simulink model "controlMCUSlugsMKII"  (Simulink 6.6)
settings: Solver=FixedStepDiscrete  StartTime=0.0  StopTime=10.0  FixedStep=0.01  RelTol=1e-3
InitFcn:
  | mcuInit
values from neighbouring files (symbols this model uses):
  apSampleTime = 0.01    [mcuInit.m]
  derivativesConstant = 5    [mcuInit.m]
  T = 0.01    [mcuInit.m]
undefined symbols (not defined in the file or in its folder): bankCommandLimit, baseHeight, bda, bde, bdr, bdt, bICda, bICde, bICdr, bICdt, controlMCUInit, daLimit, deLimit, drLimit, dtLimit, getAccBias, getAccels, getAttitude, getMidLevelCommands, getPassValues, getPidIdx, getVned, getWP, getXYZ, gsRead, ISA_g, lowRateTelemetryMavlink, mda, mde, mdr, mdt, mICda, mICde, mICdr, mICdt, pitchCommandLimit, protDecodeMavlink, readIpc, send2GS, setCurrentCommands, setDiagnosticFloat, setDiagnosticShort, setLogFloat1, setLogFloat2, setNavLat, setNavLong, setNavNav, u1, u2, updateEuler, updateLoad, updatePQR, updatePWM, updatePWM2, y1
libraries: dsPICdrivers x85, simulink x79, SLUGS_Library x23, aerolibconvert2 x5, aerolibutil x3
(part 2 of 5)

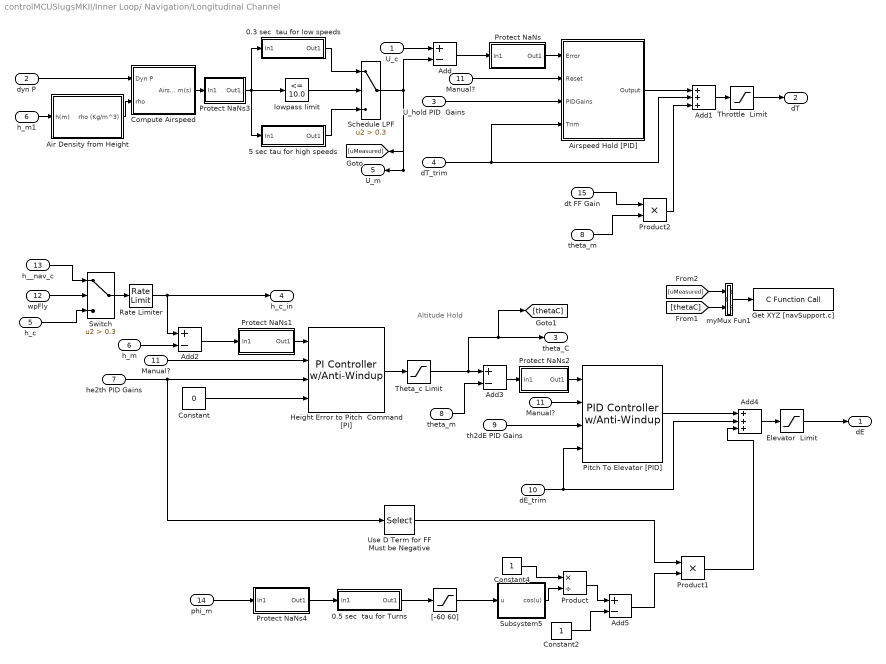
== system controlMCUSlugsMKII/Inner Loop/ Navigation/Longitudinal Channel ==
  note: Altitude Hold
  U_c : Inport
  dyn P : Inport  Port=2
  U_hold PID  Gains : Inport  Port=3
  dT_trim : Inport  Port=4
  h_c : Inport  Port=5
  h_m : Inport  Port=6
  he2th PID Gains : Inport  Port=7
  theta_m : Inport  Port=8
  th2dE PID Gains : Inport  Port=9
  dE_trim : Inport  Port=10
  Manual? : Inport  Port=11
  wpFly : Inport  Port=12  SampleTime=apSampleTime
  h__nav_c : Inport  Port=13
  phi_m : Inport  Port=14
  dt FF Gain : Inport  Port=15
  0.3 sec  tau for low speeds : Subsystem  mask(Tustin1stOrderLowpassAutoInitialCondition){f=0.5, T=T}
      mask prompts: f "Lowpass Frequency"; T "Sample Time"
      mask help: Takes a 3db rolloff frequency (in Hz, NOT radians/s) and a sample time. Performs a symbolic Tustin conversion and implements in a discrete filter. The initial output of the filter is set by the first sample.
      mask Help: Enter the desired 3db rolloff frequency in Hz and the sample time. Initial conditions are sampled automatically.
      mask Display: fprintf('%.2f Hz lowpass',f)
  0.5 sec  tau for Turns : Subsystem  mask(Tustin1stOrderLowpassAutoInitialCondition){f=0.32, T=T}
      mask prompts: f "Lowpass Frequency"; T "Sample Time"
      mask help: Takes a 3db rolloff frequency (in Hz, NOT radians/s) and a sample time. Performs a symbolic Tustin conversion and implements in a discrete filter. The initial output of the filter is set by the first sample.
      mask Help: Enter the desired 3db rolloff frequency in Hz and the sample time. Initial conditions are sampled automatically.
      mask Display: fprintf('%.2f Hz lowpass',f)
  5 sec tau for high speeds : Subsystem  mask(Tustin1stOrderLowpassAutoInitialCondition){f=.032, T=T}
      mask prompts: f "Lowpass Frequency"; T "Sample Time"
      mask help: Takes a 3db rolloff frequency (in Hz, NOT radians/s) and a sample time. Performs a symbolic Tustin conversion and implements in a discrete filter. The initial output of the filter is set by the first sample.
      mask Help: Enter the desired 3db rolloff frequency in Hz and the sample time. Initial conditions are sampled automatically.
      mask Display: fprintf('%.2f Hz lowpass',f)
  Add : Sum  Inputs=+-  OutScaling=2^-10
  Add1 : Sum  Inputs=3  OutDataTypeMode=single  OutScaling=2^-10
  Add2 : Sum  Inputs=+-  OutDataTypeMode=single  OutScaling=2^-10
  Add3 : Sum  Inputs=+-  OutDataTypeMode=single  OutScaling=2^-10
  Add4 : Sum  Inputs=3  OutDataTypeMode=single  OutScaling=2^-10
  Add5 : Sum  Inputs=+-  OutDataTypeMode=single  OutScaling=2^-10
  Air Density from Height : Subsystem  AncestorBlock=SLUGS_Library/Air Density from Height
  Airspeed Hold [PID] : Subsystem  AncestorBlock=SLUGS_Library/Control Blocks/PID Controller w//Anti-Windup  mask(PID){Tsample=apSampleTime, Ndelay=derivativesConstant, upperSaturationLimit=dtLimit, lowerSaturationLimit=0}
      mask prompts: Tsample "Sample Time"; Ndelay "Integer delays for de/dt"; upperSaturationLimit "Upper Saturation Limit"; lowerSaturationLimit "Lower Saturation Limit"
      mask help: PID controller block with anti-windup and saturation limits. Implemented as a discrete forwardl integration which stops integrating when the output is saturated. Derivative is implemented as a numerical derivative with N integer delays to smooth output.
      mask Display:
      | disp('PID')
      | port_label('input',1,'error')
      | port_label('input',3,'gains')
      | port_label('input',2,'reset')
      | port_label('input',4,'trim')
      | port_label('output',1,'output')
  Compute Airspeed : Subsystem  AncestorBlock=SLUGS_Library/Compute Airspeed
  Constant : Constant  Value=0
  Constant2 : Constant  OutDataTypeMode=single
  Constant4 : Constant  OutDataTypeMode=single
  Elevator  Limit : Saturate  UpperLimit=deLimit  LowerLimit=-deLimit  SampleTime=apSampleTime
  Get XYZ [navSupport.c] : dsPICdrivers/OTHERS/C Function Call  Tag=dsPIC_dsPIC_CFunctionCall  fctName='setNavLong'  INPUT_SIZE=2  INPUT1=real32  INPUT2=--  INPUT3=--  OUTPUT_SIZE=1  OUTPUT1=--  SampleTime=.01  InputType=[ 7 ]  OutputType=[ ]  FctDeclaration=extern void setNavLong(real32_T* u1);  FctCall=setNavLong(*%u1);  OrderingInOutPopup=None
  Height Error to Pitch  Command [PI] : SLUGS_Library/Control Blocks/PI Controller w//Anti-Windup  SystemSampleTime=-1  Tsample=apSampleTime  Ndelay=derivativesConstant  upperSaturationLimit=pitchCommandLimit  lowerSaturationLimit=-pitchCommandLimit
  "Manual? " : InportShadow  Port=11  LatchByCopyingInsideSignal=off
  "Manual?  " : InportShadow  Port=11  LatchByCopyingInsideSignal=off
  Pitch To Elevator [PID] : SLUGS_Library/Control Blocks/PID Controller w//Anti-Windup  SystemSampleTime=-1  Tsample=apSampleTime  Ndelay=derivativesConstant  upperSaturationLimit=deLimit  lowerSaturationLimit=-deLimit
  Product : Product  Inputs=*/  RndMeth=Zero
  Product1 : Product  RndMeth=Zero
  Product2 : Product  RndMeth=Zero
  Protect NaNs : Subsystem
  Protect NaNs1 : Subsystem
  Protect NaNs2 : Subsystem
  Protect NaNs3 : Subsystem
  Protect NaNs4 : Subsystem
  Rate Limiter : RateLimiter  RisingSlewLimit=7  FallingSlewLimit=-5  SampleTimeMode=inherited  InitialCondition=baseHeight
  Schedule LPF : Switch  Criteria=u2 > Threshold  Threshold=0.3
  Subsystem5 : Subsystem  AncestorBlock=SLUGS_Library/Subsystem5
  Switch : Switch  Criteria=u2 > Threshold  Threshold=0.3  InputSameDT=on
  Theta_c Limit : Saturate  UpperLimit=pitchCommandLimit  LowerLimit=-pitchCommandLimit  SampleTime=apSampleTime
  Throttle  Limit : Saturate  UpperLimit=dtLimit  LowerLimit=0  SampleTime=apSampleTime
  Use D Term for FF Must be Negative : Selector  IndexOptions=Index vector (dialog)  Indices=3  OutputSizes=1  InputPortWidth=3
  "[-60 60]" : Saturate  UpperLimit=60  LowerLimit=-60  SampleTime=apSampleTime
  h_m1 : InportShadow  Port=6  LatchByCopyingInsideSignal=off
  lowpass limit : simulink/Logic and Bit Operations/Compare To Constant  SystemSampleTime=-1  relop=<=  const=10.0  LogicOutDataTypeMode=uint8  ZeroCross=off
  myMux Fun1 : Stateflow chart
  "theta_m " : InportShadow  Port=8  LatchByCopyingInsideSignal=off
  dE : Outport
  dT : Outport  Port=2
  theta_C : Outport  Port=3
  h_c_in : Outport  Port=4
  U_m : Outport  Orientation=left  Port=5
  wires:
  Height Error to Pitch  Command [PI]/1 -> Theta_c Limit/1
  Rate Limiter/1 -> Add2/1, h_c_in/1
  h__nav_c/1 -> Switch/1
  h_c/1 -> Switch/3
  Switch/1 -> Rate Limiter/1
  wpFly/1 -> Switch/2
  Theta_c Limit/1 -> Add3/1, theta_C/1, [thetaC]
  Add3/1 -> Protect NaNs2/1(In1)
  th2dE PID Gains/1 -> Pitch To Elevator [PID]/3
  he2th PID Gains/1 -> Use D Term for FF Must be Negative/1, Height Error to Pitch  Command [PI]/3
  h_m1/1 -> Air Density from Height/1(h(m))
  dyn P/1 -> Compute Airspeed/1(Dyn P)
  Air Density from Height/1(rho (Kg/m^3)) -> Compute Airspeed/2(rho)
  Elevator  Limit/1 -> dE/1
  dE_trim/1 -> Add4/2, Pitch To Elevator [PID]/4
  Pitch To Elevator [PID]/1 -> Add4/1
  Add4/1 -> Elevator  Limit/1
  "Manual?  "/1 -> Pitch To Elevator [PID]/2
  "Manual? "/1 -> Height Error to Pitch  Command [PI]/2
  Manual?/1 -> Airspeed Hold [PID]/2(Reset)
  theta_m/1 -> Add3/2
  h_m/1 -> Add2/2
  Add2/1 -> Protect NaNs1/1(In1)
  Throttle  Limit/1 -> dT/1
  Add1/1 -> Throttle  Limit/1
  dT_trim/1 -> Add1/2, Airspeed Hold [PID]/4(Trim)
  Airspeed Hold [PID]/1(Output) -> Add1/1
  Add/1 -> Protect NaNs/1(In1)
  U_c/1 -> Add/1
  myMux Fun1/1(y) -> Get XYZ [navSupport.c]/1
  [uMeasured] -> myMux Fun1/1(u1)
  [thetaC] -> myMux Fun1/2(u2)
  Schedule LPF/1 -> Add/2, U_m/1, [uMeasured]
  Compute Airspeed/1(Airspeed m(s)) -> Protect NaNs3/1(In1)
  lowpass limit/1 -> Schedule LPF/2
  5 sec tau for high speeds/1(Out1) -> Schedule LPF/3
  0.3 sec  tau for low speeds/1(Out1) -> Schedule LPF/1
  phi_m/1 -> Protect NaNs4/1(In1)
  Constant2/1 -> Add5/2
  Subsystem5/1(cos(u)) -> Product/2
  Constant4/1 -> Product/1
  Product/1 -> Add5/1
  0.5 sec  tau for Turns/1(Out1) -> "[-60 60]"/1
  "[-60 60]"/1 -> Subsystem5/1(u)
  Add5/1 -> Product1/2
  Use D Term for FF Must be Negative/1 -> Product1/1
  Product1/1 -> Add4/3
  "theta_m "/1 -> Product2/2
  Product2/1 -> Add1/3
  dt FF Gain/1 -> Product2/1
  U_hold PID  Gains/1 -> Airspeed Hold [PID]/3(PIDGains)
  Constant/1 -> Height Error to Pitch  Command [PI]/4
  Protect NaNs/1(Out1) -> Airspeed Hold [PID]/1(Error)
  Protect NaNs1/1(Out1) -> Height Error to Pitch  Command [PI]/1
  Protect NaNs2/1(Out1) -> Pitch To Elevator [PID]/1
  Protect NaNs3/1(Out1) -> 0.3 sec  tau for low speeds/1(In1), 5 sec tau for high speeds/1(In1), lowpass limit/1
  Protect NaNs4/1(Out1) -> 0.5 sec  tau for Turns/1(In1)

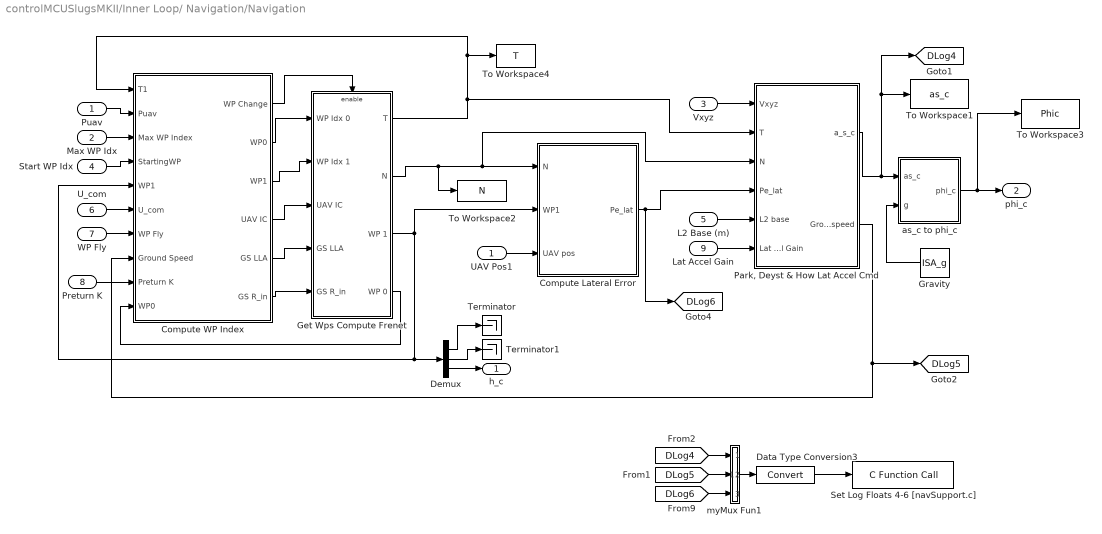
== system controlMCUSlugsMKII/Inner Loop/ Navigation/Navigation ==
  Puav : Inport  SampleTime=apSampleTime
  Max WP Idx : Inport  Port=2
  Vxyz : Inport  Port=3
  Start WP Idx : Inport  Port=4
  L2 Base (m) : Inport  Port=5
  U_com : Inport  Port=6
  WP Fly : Inport  Port=7
  Preturn K : Inport  Port=8
  Lat Accel Gain : Inport  Port=9
  Compute Lateral Error : Subsystem  AncestorBlock=SLUGS_Library/Navigation/Compute Lateral Error
  Compute WP Index : Subsystem
  Data Type Conversion3 : DataTypeConversion  OutDataTypeMode=single
  Demux : Demux  Outputs=3
  Get Wps Compute Frenet : Subsystem
  Gravity : Constant  Orientation=left  Value=ISA_g  OutDataTypeMode=single
  "Park, Deyst & How Lat Accel Cmd" : Subsystem  AncestorBlock=SLUGS_Library/Navigation/Park, Deyst & How Lat Accel Cmd
  Set Log Floats 4-6 [navSupport.c] : dsPICdrivers/OTHERS/C Function Call  Tag=dsPIC_dsPIC_CFunctionCall  fctName='setLogFloat2'  INPUT_SIZE=3  INPUT1=real32  INPUT2=--  INPUT3=--  OUTPUT_SIZE=1  OUTPUT1=--  SampleTime=.01  InputType=[ 7 ]  OutputType=[ ]  FctDeclaration=extern void setLogFloat2(real32_T* u1);  FctCall=setLogFloat2(*%u1);  OrderingInOutPopup=None
  Terminator : Terminator
  Terminator1 : Terminator
  To Workspace1 : ToWorkspace  VariableName=as_c  SampleTime=-1  SaveFormat=Array
  To Workspace2 : ToWorkspace  VariableName=N  SampleTime=-1  SaveFormat=Array
  To Workspace3 : ToWorkspace  VariableName=Phic  SampleTime=-1  SaveFormat=Array
  To Workspace4 : ToWorkspace  VariableName=T  SampleTime=-1  SaveFormat=Array
  UAV Pos1 : InportShadow  Port=1  SampleTime=apSampleTime  LatchByCopyingInsideSignal=off
  as_c to phi_c : Subsystem  AncestorBlock=SLUGS_Library/Navigation/as_c to phi_c
  myMux Fun1 : Stateflow chart
  h_c : Outport
  phi_c : Outport  Port=2
  tag scope: DLog4=global, DLog5=global, DLog6=global
  wires:
  Demux/2 -> Terminator1/1
  Demux/1 -> Terminator/1
  Demux/3 -> h_c/1
  Compute WP Index/6(GS R_in) -> Get Wps Compute Frenet/5(GS R_in)
  Compute WP Index/5(GS LLA) -> Get Wps Compute Frenet/4(GS LLA)
  Compute WP Index/2(WP0) -> Get Wps Compute Frenet/1(WP Idx 0)
  Compute WP Index/3(WP1) -> Get Wps Compute Frenet/2(WP Idx 1)
  Get Wps Compute Frenet/2(N) -> Compute Lateral Error/1(N), "Park, Deyst & How Lat Accel Cmd"/3(N), To Workspace2/1
  Get Wps Compute Frenet/1(T) -> To Workspace4/1, Compute WP Index/1(T1), "Park, Deyst & How Lat Accel Cmd"/2(T)
  Puav/1 -> Compute WP Index/2(Puav)
  Max WP Idx/1 -> Compute WP Index/3(Max WP Index)
  Start WP Idx/1 -> Compute WP Index/4(StartingWP)
  "Park, Deyst & How Lat Accel Cmd"/1(a_s_c) -> as_c to phi_c/1(as_c), To Workspace1/1, [DLog4]
  UAV Pos1/1 -> Compute Lateral Error/3(UAV pos)
  as_c to phi_c/1(phi_c) -> phi_c/1, To Workspace3/1
  Gravity/1 -> as_c to phi_c/2(g)
  Compute Lateral Error/1(Pe_lat) -> "Park, Deyst & How Lat Accel Cmd"/4(Pe_lat), [DLog6]
  Get Wps Compute Frenet/3(WP 1) -> Compute Lateral Error/2(WP1), Demux/1, Compute WP Index/5("WP1 ")
  L2 Base (m)/1 -> "Park, Deyst & How Lat Accel Cmd"/5(L2 base)
  Compute WP Index/1(WP Change) -> Get Wps Compute Frenet/Enable
  U_com/1 -> Compute WP Index/6(U_com)
  Vxyz/1 -> "Park, Deyst & How Lat Accel Cmd"/1(Vxyz)
  WP Fly/1 -> Compute WP Index/7(WP Fly)
  Compute WP Index/4(UAV IC) -> Get Wps Compute Frenet/3(UAV IC)
  "Park, Deyst & How Lat Accel Cmd"/2(Groundspeed) -> Compute WP Index/8(Ground Speed), [DLog5]
  Preturn K/1 -> Compute WP Index/9(Preturn K)
  Get Wps Compute Frenet/4(WP 0) -> Compute WP Index/10("WP0 ")
  Lat Accel Gain/1 -> "Park, Deyst & How Lat Accel Cmd"/6(Lat Accel Gain)
  [DLog4] -> myMux Fun1/1(u1)
  [DLog5] -> myMux Fun1/2(u2)
  [DLog6] -> myMux Fun1/3(u3)
  myMux Fun1/1(y) -> Data Type Conversion3/1
  Data Type Conversion3/1 -> Set Log Floats 4-6 [navSupport.c]/1

== system controlMCUSlugsMKII/Inner Loop/ Navigation/Protect NaNs ==
  In1 : Inport
  Integer Delay3 : simulink/Discrete/Integer Delay  Orientation=left  vinit=0.0  samptime=T  NumDelays=1
  Relational Operator2 : RelationalOperator  Operator===  LogicOutDataTypeMode=Specify via dialog
  Switch3 : Switch  Criteria=u2 > Threshold  Threshold=0.3  SampleTime=.01
  Out1 : Outport  Orientation=down
  wires:
  Integer Delay3/1 -> Switch3/3
  Switch3/1 -> Out1/1, Integer Delay3/1
  In1/1 -> Relational Operator2/2, Relational Operator2/1, Switch3/1
  Relational Operator2/1 -> Switch3/2

== system controlMCUSlugsMKII/Trim Vals/Bufffer IC ==
  Pilot Console : Inport
  Buffer IC Channel : Stateflow chart
  Buffer IC Channel1 : Stateflow chart
  Buffer IC Channel2 : Stateflow chart
  Buffer IC Channel3 : Stateflow chart
  Demux : Demux
  dT_buf : Outport
  dA_buf : Outport  Port=2
  dR_buf : Outport  Port=3
  dE_buf : Outport  Port=4
  wires:
  Demux/1 -> Buffer IC Channel/1(latest)
  Demux/2 -> Buffer IC Channel1/1(latest)
  Demux/3 -> Buffer IC Channel2/1(latest)
  Demux/4 -> Buffer IC Channel3/1(latest)
  Pilot Console/1 -> Demux/1
  Buffer IC Channel/1(history) -> dT_buf/1
  Buffer IC Channel1/1(history) -> dA_buf/1
  Buffer IC Channel2/1(history) -> dR_buf/1
  Buffer IC Channel3/1(history) -> dE_buf/1

== system controlMCUSlugsMKII/Trim Vals/Control Surface Input ==
  Input Capture : dsPICdrivers/Peripheral I//O/Input Capture  Tag=dsPIC_PWM_IC  Priority=5  IntPriority=6  Channel=[ 2 3 4 5 8]  Channel_UP_Down_Periode="[1  1  1  1  1]"  MaxChannel="[0.0025      0.0025      0.0025      0.0025      0.0025]"  SafeMarge="[10  10  10  10  10]"  MaxName=' IC2max , IC3max , IC4max , IC5max , IC8max '  Precision="[13.7469      13.7469      13.7469      13.7469      13.7469]"  Timer="[2  2  2  2  2]"  ChangeDetected="[0  0  0  0  0]"  ChangeDetectedPortRef=3  SampleTime=.01  Status=OK
  myMux Fun5 : Stateflow chart
  Pilot Console : Outport
  wires:
  myMux Fun5/1(y) -> Pilot Console/1
  Input Capture/1 -> myMux Fun5/1(u1)
  Input Capture/2 -> myMux Fun5/2(u2)
  Input Capture/3 -> myMux Fun5/3(u3)
  Input Capture/4 -> myMux Fun5/4(u4)
  Input Capture/5 -> myMux Fun5/5(u5)

== system controlMCUSlugsMKII/Trim Vals/Detect Transition High to Low ==
  Switch : Inport
  Add : Sum  Orientation=left  Inputs=2  OutDataTypeMode=uint8  OutScaling=2^-10
  Data Type Conversion : DataTypeConversion  OutDataTypeMode=double  SampleTime=apSampleTime
  Hit  Crossing : HitCross  HitCrossingOffset=0.5  HitCrossingDirection=falling  SampleTime=apSampleTime
  IC : InitialCondition  Orientation=down
  Integer Delay2 : simulink/Discrete/Integer Delay  Orientation=left  vinit=0  samptime=-1  NumDelays=1
  Transition : Outport  Orientation=left
  wires:
  Hit  Crossing/1 -> IC/1
  Data Type Conversion/1 -> Hit  Crossing/1
  Integer Delay2/1 -> Add/1
  IC/1 -> Add/2, Integer Delay2/1
  Switch/1 -> Data Type Conversion/1
  Add/1 -> Transition/1

== system controlMCUSlugsMKII/Trim Vals/Grab I.C. ==
  dT_buf : Inport
  dA_buf : Inport  Port=2
  dR_buf : Inport  Port=3
  dE_buf : Inport  Port=4
  U_m : Inport  Port=5
  Enable : EnablePort
  Choose the Median [navSupport.c]{,1..3} (4 alike) : dsPICdrivers/OTHERS/C Function Call  Tag=dsPIC_dsPIC_CFunctionCall  fctName='meanFilter5'  INPUT_SIZE=7  INPUT1=uint16  INPUT2=--  INPUT3=--  OUTPUT_SIZE=1  OUTPUT1=uint16  SampleTime=.01  InputType=[ 4 ]  OutputType=[ 4 ]  FctDeclaration=extern uint16_T meanFilter5(uint16_T* u1);  FctCall=%y1 = meanFilter5(*%u1);  OrderingInOutPopup=None
  Convert to Rad : Subsystem  mask{slopem=mICdt, interceptb=bICdt}
      mask prompts: slopem "Slope"; interceptb "Intercept"
  Convert to Rad1 : Subsystem  mask{slopem=mICda, interceptb=bICda}
      mask prompts: slopem "Slope"; interceptb "Intercept"
  Convert to Rad2 : Subsystem  mask{slopem=mICdr, interceptb=bICdr}
      mask prompts: slopem "Slope"; interceptb "Intercept"
  Convert to Rad3 : Subsystem  mask{slopem=mICde, interceptb=bICde}
      mask prompts: slopem "Slope"; interceptb "Intercept"
  Set Current Height and Airspeed as Commands [navSupport.c] : dsPICdrivers/OTHERS/C Function Call  Tag=dsPIC_dsPIC_CFunctionCall  fctName='setCurrentCommands'  INPUT_SIZE=1  INPUT1=real32  INPUT2=--  INPUT3=--  OUTPUT_SIZE=1  OUTPUT1=--  SampleTime=.01  InputType=[ 7 ]  OutputType=[ ]  FctDeclaration=extern void setCurrentCommands(real32_T u1);  FctCall=setCurrentCommands(%u1);  OrderingInOutPopup=None
  dT_trim : Outport
  dA_trim : Outport  Port=2
  dR_trim : Outport  Port=3
  dE_trim : Outport  Port=4
  wires:
  U_m/1 -> Set Current Height and Airspeed as Commands [navSupport.c]/1
  Convert to Rad/1(Angle (rad)) -> dT_trim/1
  Convert to Rad1/1(Angle (rad)) -> dA_trim/1
  Convert to Rad2/1(Angle (rad)) -> dR_trim/1
  Convert to Rad3/1(Angle (rad)) -> dE_trim/1
  Choose the Median [navSupport.c]/1 -> Convert to Rad/1(IC)
  Choose the Median [navSupport.c]1/1 -> Convert to Rad1/1(IC)
  Choose the Median [navSupport.c]2/1 -> Convert to Rad2/1(IC)
  Choose the Median [navSupport.c]3/1 -> Convert to Rad3/1(IC)
  dT_buf/1 -> Choose the Median [navSupport.c]/1
  dA_buf/1 -> Choose the Median [navSupport.c]1/1
  dR_buf/1 -> Choose the Median [navSupport.c]2/1
  dE_buf/1 -> Choose the Median [navSupport.c]3/1

== system controlMCUSlugsMKII/Trim Vals/Log  Trims Using PWM High [groundStationDriver.c] ==
  In1 : Inport
  In2 : Inport  Port=2
  In3 : Inport  Port=3
  In4 : Inport  Port=4
  Data Type Conversion{1..4} (4 alike) : DataTypeConversion  OutDataTypeMode=uint16  SampleTime=apSampleTime
  Report Airspeed : Subsystem
  Update PWM  Commands1 [updateControlMcu.c] : dsPICdrivers/OTHERS/C Function Call  Tag=dsPIC_dsPIC_CFunctionCall  fctName='updatePWM2'  INPUT_SIZE=1  INPUT1=uint16  INPUT2=uint8  INPUT3=--  OUTPUT_SIZE=1  OUTPUT1=--  SampleTime=-1  InputType=[ 4 2 ]  OutputType=[ ]  FctDeclaration=extern void updatePWM2(uint16_T u1, uint8_T u2);  FctCall=updatePWM2(%u1, %u2);  OrderingInOutPopup=None
  Update PWM  Commands2 [updateControlMcu.c] : dsPICdrivers/OTHERS/C Function Call  Tag=dsPIC_dsPIC_CFunctionCall  fctName='updatePWM2'  INPUT_SIZE=1  INPUT1=uint16  INPUT2=uint8  INPUT3=--  OUTPUT_SIZE=1  OUTPUT1=--  SampleTime=-1  InputType=[ 4 2 ]  OutputType=[ ]  FctDeclaration=extern void updatePWM2(uint16_T u1, uint8_T u2);  FctCall=updatePWM2(%u1, %u2);  OrderingInOutPopup=None
  Update PWM  Commands3 [updateControlMcu.c] : dsPICdrivers/OTHERS/C Function Call  Tag=dsPIC_dsPIC_CFunctionCall  fctName='updatePWM2'  INPUT_SIZE=1  INPUT1=uint16  INPUT2=uint8  INPUT3=--  OUTPUT_SIZE=1  OUTPUT1=--  SampleTime=-1  InputType=[ 4 2 ]  OutputType=[ ]  FctDeclaration=extern void updatePWM2(uint16_T u1, uint8_T u2);  FctCall=updatePWM2(%u1, %u2);  OrderingInOutPopup=None
  Update PWM  Commands4 [updateControlMcu.c] : dsPICdrivers/OTHERS/C Function Call  Tag=dsPIC_dsPIC_CFunctionCall  fctName='updatePWM2'  INPUT_SIZE=1  INPUT1=uint16  INPUT2=uint8  INPUT3=--  OUTPUT_SIZE=1  OUTPUT1=--  SampleTime=-1  InputType=[ 4 2 ]  OutputType=[ ]  FctDeclaration=extern void updatePWM2(uint16_T u1, uint8_T u2);  FctCall=updatePWM2(%u1, %u2);  OrderingInOutPopup=None
  dlf : Constant  OutDataTypeMode=uint8
  dlf1 : Constant  Value=3  OutDataTypeMode=uint8
  dre : Constant  Value=0  OutDataTypeMode=uint8
  dre1 : Constant  Value=2  OutDataTypeMode=uint8
  wires:
  Data Type Conversion3/1 -> Update PWM  Commands2 [updateControlMcu.c]/1
  In2/1 -> Data Type Conversion3/1
  dlf/1 -> Update PWM  Commands2 [updateControlMcu.c]/2
  Data Type Conversion1/1 -> Update PWM  Commands3 [updateControlMcu.c]/1
  Data Type Conversion4/1 -> Update PWM  Commands4 [updateControlMcu.c]/1
  In3/1 -> Data Type Conversion1/1
  In4/1 -> Data Type Conversion4/1
  dre1/1 -> Update PWM  Commands3 [updateControlMcu.c]/2
  dlf1/1 -> Update PWM  Commands4 [updateControlMcu.c]/2
  Data Type Conversion2/1 -> Update PWM  Commands1 [updateControlMcu.c]/1
  dre/1 -> Update PWM  Commands1 [updateControlMcu.c]/2
  In1/1 -> Data Type Conversion2/1

== system controlMCUSlugsMKII/Update PWM Commands and Send Telemetry/Generate PWM Signals Based on the Control Type ==
  Ctrl Type : Inport
  PWM(rad) : Inport  Port=2
  Pilot Console (IC) : Inport  Port=3
  Data Type Conversion : DataTypeConversion  OutDataTypeMode=uint16
  If : If  IfExpression=u1 == 1  ElseIfExpressions=((u1 == 2 ) | (u1 == 3)), u1 == 4, u1 == 5  ShowElse=off  SampleTime=.01
  If  Control Type Is Manual : Subsystem  TreatAsAtomicUnit=on
  If  Control Type Is Passthrough : Subsystem  TreatAsAtomicUnit=on
  If  Control Type Is Selective Passthrough : Subsystem  TreatAsAtomicUnit=on
  If  Control Type Is Wp Follow  or Inner Cmds : Subsystem  TreatAsAtomicUnit=on
  Merge : Merge  Inputs=4
  PWM : Outport
  wires:
  If/1 -> If  Control Type Is Manual/Action
  If/2 -> If  Control Type Is Wp Follow  or Inner Cmds/Action
  If/3 -> If  Control Type Is Passthrough/Action
  If/4 -> If  Control Type Is Selective Passthrough/Action
  If  Control Type Is Manual/1(PWM) -> Merge/1
  If  Control Type Is Wp Follow  or Inner Cmds/1(PWM (abs)) -> Merge/2
  If  Control Type Is Passthrough/1(PWM (abs)) -> Merge/3
  If  Control Type Is Selective Passthrough/1(PWM) -> Merge/4
  PWM(rad)/1 -> If  Control Type Is Selective Passthrough/1(PWM(rad)), If  Control Type Is Wp Follow  or Inner Cmds/1(PWM(rad))
  Pilot Console (IC)/1 -> If  Control Type Is Passthrough/1(Pilot (IC)), If  Control Type Is Selective Passthrough/2(Pilot (IC)), If  Control Type Is Manual/1(Pilot (IC))
  Ctrl Type/1 -> If/1
  Merge/1 -> Data Type Conversion/1
  Data Type Conversion/1 -> PWM/1

== system controlMCUSlugsMKII/get Nav Vars/Direction Cosine Matrix to Euler Angles ==
  DCM : Inport  PortDimensions=[3,3]
  "Reshape 3x3 -> 9" : Reshape  OutputDimensions=[9, 1]
  Subsystem1 : Subsystem  AncestorBlock=SLUGS_Library/Subsystem4
  Subsystem2 : Subsystem  AncestorBlock=SLUGS_Library/Subsystem4
  Subsystem3 : Subsystem  AncestorBlock=SLUGS_Library/Subsystem6
  cos(phi)cos(theta) : Subsystem
  cos(psi)cos(theta) : Subsystem
  sin(phi)cos(theta) : Subsystem
  sin(psi)cos(theta) : Subsystem
  sin(theta) : Subsystem
  phi : Outport  PortDimensions=1  InitialOutput=0
  theta : Outport  Port=2  PortDimensions=1  InitialOutput=0
  psi : Outport  Port=3  PortDimensions=1  InitialOutput=0
  wires:
  DCM/1 -> "Reshape 3x3 -> 9"/1
  "Reshape 3x3 -> 9"/1 -> sin(theta)/1(DCM), cos(phi)cos(theta)/1(DCM), sin(phi)cos(theta)/1(DCM), cos(psi)cos(theta)/1(DCM), sin(psi)cos(theta)/1(DCM)
  sin(theta)/1(sin(theta)) -> Subsystem3/1(x)
  sin(phi)cos(theta)/1(sin(phi)cos(theta)) -> Subsystem2/1(u)
  cos(phi)cos(theta)/1(cos(phi)cos(theta)) -> Subsystem2/2(v)
  sin(psi)cos(theta)/1(sin(psi)cos(theta)) -> Subsystem1/1(u)
  cos(psi)cos(theta)/1(cos(psi)cos(theta)) -> Subsystem1/2(v)
  Subsystem2/1(atan2(x,y)) -> phi/1  "phi"
  Subsystem3/1(asin(x)) -> theta/1  "theta"
  Subsystem1/1(atan2(x,y)) -> psi/1  "psi"

== system controlMCUSlugsMKII/get Nav Vars/Euler Angles to  Direction Cosine Matrix1 ==
  Euler Roll Pitch Yaw : Inport  PortDimensions=3
  A11 : Subsystem
  A12 : Subsystem
  A13 : Subsystem
  A21 : Subsystem
  A22 : Subsystem
  A23 : Subsystem
  A31 : Subsystem
  A32 : Subsystem
  A33 : Subsystem
  Create Transformation Matrix : Subsystem  AncestorBlock=aerolibutil/Create 3x3 Matrix  mask(Create 3x3 Matrix){}
      mask help:
      | Create a 3-by-3 matrix from nine input values. Each input corresponds to an element of the matrix.
      |
      | For example, the input labeled A21 is the entry in the second row and first column of the matrix.
      mask init:
      | aeroicon('aeroblk');
      mask Help: web(asbhelp);
      mask Display:
      | port_label('input',1,'A_{11}','texmode','on');
      | port_label('input',2,'A_{12}','texmode','on');
      | port_label('input',3,'A_{13}','texmode','on');
      | port_label('input',4,'A_{21}','texmode','on');
      | port_label('input',5,'A_{22}','texmode','on');
      | port_label('input',6,'A_{23}','texmode','on');
      | port_label('input',7,'A_{31}','texmode','on');
      | port_label('input',8,'A_{32}','texmode','on');
      | port_label('input',9,'A_{33}','texmode','on');
      | port_label('output',1,'A','texmode','on');
  Mux : Mux  Inputs=2
  Subsystem5 : Subsystem  AncestorBlock=SLUGS_Library/Subsystem5
  DCM : Outport  PortDimensions=[3,3]  InitialOutput=0
  wires:
  Mux/1 -> A33/1(sin_cos), A32/1(sin_cos), A31/1(sin_cos), A23/1(sin_cos), A13/1(sin_cos), A11/1(sin_cos), A12/1(sin_cos), A21/1(sin_cos), A22/1(sin_cos)
  Euler Roll Pitch Yaw/1 -> Subsystem5/1(u)
  Subsystem5/2(cos(u)) -> Mux/2
  Subsystem5/1(sin(u)) -> Mux/1
  Create Transformation Matrix/1(Matrix) -> DCM/1
  A21/1(A21) -> Create Transformation Matrix/4(M21)
  A31/1(A31) -> Create Transformation Matrix/7(M31)
  A32/1(A32) -> Create Transformation Matrix/8(M32)
  A33/1(A33) -> Create Transformation Matrix/9(M33)
  A23/1(A23) -> Create Transformation Matrix/6(M23)
  A12/1(A12) -> Create Transformation Matrix/2(M12)
  A11/1(A11) -> Create Transformation Matrix/1(M11)
  A22/1(A22) -> Create Transformation Matrix/5(M22)
  A13/1(A13) -> Create Transformation Matrix/3(M13)

== system controlMCUSlugsMKII/get Nav Vars/Euler Angles to  Direction Cosine Matrix2 ==
  Euler Roll Pitch Yaw : Inport  PortDimensions=3
  A11 : Subsystem
  A12 : Subsystem
  A13 : Subsystem
  A21 : Subsystem
  A22 : Subsystem
  A23 : Subsystem
  A31 : Subsystem
  A32 : Subsystem
  A33 : Subsystem
  Create Transformation Matrix : Subsystem  AncestorBlock=aerolibutil/Create 3x3 Matrix  mask(Create 3x3 Matrix){}
      mask help:
      | Create a 3-by-3 matrix from nine input values. Each input corresponds to an element of the matrix.
      |
      | For example, the input labeled A21 is the entry in the second row and first column of the matrix.
      mask init:
      | aeroicon('aeroblk');
      mask Help: web(asbhelp);
      mask Display:
      | port_label('input',1,'A_{11}','texmode','on');
      | port_label('input',2,'A_{12}','texmode','on');
      | port_label('input',3,'A_{13}','texmode','on');
      | port_label('input',4,'A_{21}','texmode','on');
      | port_label('input',5,'A_{22}','texmode','on');
      | port_label('input',6,'A_{23}','texmode','on');
      | port_label('input',7,'A_{31}','texmode','on');
      | port_label('input',8,'A_{32}','texmode','on');
      | port_label('input',9,'A_{33}','texmode','on');
      | port_label('output',1,'A','texmode','on');
  Mux : Mux  Inputs=2
  Subsystem5 : Subsystem  AncestorBlock=SLUGS_Library/Subsystem5
  DCM : Outport  PortDimensions=[3,3]  InitialOutput=0
  wires:
  A13/1(A13) -> Create Transformation Matrix/3(M13)
  A22/1(A22) -> Create Transformation Matrix/5(M22)
  A11/1(A11) -> Create Transformation Matrix/1(M11)
  A12/1(A12) -> Create Transformation Matrix/2(M12)
  A23/1(A23) -> Create Transformation Matrix/6(M23)
  A33/1(A33) -> Create Transformation Matrix/9(M33)
  A32/1(A32) -> Create Transformation Matrix/8(M32)
  A31/1(A31) -> Create Transformation Matrix/7(M31)
  A21/1(A21) -> Create Transformation Matrix/4(M21)
  Create Transformation Matrix/1(Matrix) -> DCM/1
  Subsystem5/1(sin(u)) -> Mux/1
  Subsystem5/2(cos(u)) -> Mux/2
  Euler Roll Pitch Yaw/1 -> Subsystem5/1(u)
  Mux/1 -> A22/1(sin_cos), A21/1(sin_cos), A12/1(sin_cos), A11/1(sin_cos), A13/1(sin_cos), A23/1(sin_cos), A31/1(sin_cos), A32/1(sin_cos), A33/1(sin_cos)

== system controlMCUSlugsMKII/Inner Loop/ Navigation/Compute psi_dot_m/Protect NaNs ==
  In1 : Inport
  Integer Delay3 : simulink/Discrete/Integer Delay  Orientation=left  vinit=0.0  samptime=T  NumDelays=1
  Relational Operator2 : RelationalOperator  Operator===  LogicOutDataTypeMode=Specify via dialog
  Switch3 : Switch  Criteria=u2 > Threshold  Threshold=0.3  SampleTime=.01
  Out1 : Outport  Orientation=down
  wires:
  Integer Delay3/1 -> Switch3/3
  Switch3/1 -> Out1/1, Integer Delay3/1
  In1/1 -> Relational Operator2/2, Relational Operator2/1, Switch3/1
  Relational Operator2/1 -> Switch3/2

== system controlMCUSlugsMKII/Inner Loop/ Navigation/Compute psi_dot_m/Subsystem5 ==
  u : Inport
  Environment Controller1 : simulink/Signal Routing/Environment Controller  SystemSampleTime=-1
  Trigonometric Function : Trigonometry  Operator=cos
  "[apUtils.c]" : dsPICdrivers/OTHERS/C Function Call  Tag=dsPIC_dsPIC_CFunctionCall  fctName='myCos'  INPUT_SIZE=1  INPUT1=real32  INPUT2=--  INPUT3=--  OUTPUT_SIZE=1  OUTPUT1=real32  SampleTime=-1  InputType=[ 7 ]  OutputType=[ 7 ]  FctDeclaration=extern real32_T myCos(real32_T u1);  FctCall=%y1 = myCos(%u1);  OrderingInOutPopup=None
  cos(u) : Outport
  wires:
  Trigonometric Function/1 -> Environment Controller1/1
  "[apUtils.c]"/1 -> Environment Controller1/2
  Environment Controller1/1 -> cos(u)/1
  u/1 -> Trigonometric Function/1, "[apUtils.c]"/1

== system controlMCUSlugsMKII/Inner Loop/ Navigation/Compute psi_dot_m/Subsystem7 ==
  x : Inport
  Environment Controller : simulink/Signal Routing/Environment Controller  SystemSampleTime=-1
  Trigonometric Function : Trigonometry
  "[apUtils.c]" : dsPICdrivers/OTHERS/C Function Call  Tag=dsPIC_dsPIC_CFunctionCall  fctName='mySin'  INPUT_SIZE=1  INPUT1=real32  INPUT2=--  INPUT3=--  OUTPUT_SIZE=1  OUTPUT1=real32  SampleTime=-1  InputType=[ 7 ]  OutputType=[ 7 ]  FctDeclaration=extern real32_T mySin(real32_T u1);  FctCall=%y1 = mySin(%u1);  OrderingInOutPopup=None
  sin(x) : Outport
  wires:
  x/1 -> "[apUtils.c]"/1, Trigonometric Function/1
  Trigonometric Function/1 -> Environment Controller/1
  "[apUtils.c]"/1 -> Environment Controller/2
  Environment Controller/1 -> sin(x)/1

== system controlMCUSlugsMKII/Inner Loop/ Navigation/L1 Output Feedback Controller With  Projection Operator/Control  Law ==
  a : Inport
  u : Inport  Port=2
  Compute Coef : Subsystem
  Detect Change : Subsystem
  Divide : Product  OutScaling=2^-10  SampleTime=apSampleTime
  Divide1 : Product  OutScaling=2^-10  SampleTime=apSampleTime
  IC : InitialCondition
  Integer Delay : simulink/Discrete/Integer Delay  vinit=0.0  samptime=apSampleTime  NumDelays=1
  Integer Delay1 : simulink/Discrete/Integer Delay  Orientation=left  vinit=0.0  samptime=apSampleTime  NumDelays=1
  Subtract : Sum  OutScaling=2^-10  SampleTime=apSampleTime
  y : Outport
  wires:
  a/1 -> Compute Coef/1(a), Detect Change/1(Data)
  Compute Coef/1(b) -> Divide/1
  Compute Coef/2(c) -> Divide1/1
  Detect Change/1(change?) -> IC/1
  Integer Delay/1 -> Divide/2
  Divide/1 -> Subtract/1
  Divide1/1 -> Subtract/2
  Subtract/1 -> y/1, Integer Delay1/1
  IC/1 -> Compute Coef/Enable
  u/1 -> Integer Delay/1
  Integer Delay1/1 -> Divide1/2

== system controlMCUSlugsMKII/Inner Loop/ Navigation/L1 Output Feedback Controller With  Projection Operator/Projection Operator ==
  Theta Max : Inport
  Eps 0 : Inport  Port=2
  Theta : Inport  Port=3
  y : Inport  Port=4
  Compare To Zero : simulink/Logic and Bit Operations/Compare To Zero  SystemSampleTime=-1  relop=>=  LogicOutDataTypeMode=boolean  ZeroCross=off
  Compare To Zero1 : simulink/Logic and Bit Operations/Compare To Zero  SystemSampleTime=-1  relop=>  LogicOutDataTypeMode=boolean  ZeroCross=off
  Divide2 : Product  OutDataTypeMode=single  OutScaling=2^-10
  Enabled Subsystem : Subsystem  TreatAsAtomicUnit=on
  Enabled Subsystem1 : Subsystem  TreatAsAtomicUnit=on
  F(theta) : Subsystem
  Logical Operator : Logic  Operator=NOT  AllPortsSameDT=off  OutDataTypeMode=Specify via dialog
  Logical Operator2 : Logic  Orientation=down  AllPortsSameDT=off  OutDataTypeMode=Specify via dialog
  Merge : Merge  InitialOutput=0
  "y " : InportShadow  Port=4  LatchByCopyingInsideSignal=off
  "y    " : InportShadow  Port=4  LatchByCopyingInsideSignal=off
  "Proj(the, y)" : Outport
  wires:
  Theta Max/1 -> F(theta)/1(Theta Max)
  Eps 0/1 -> F(theta)/2(Eps 0)
  Theta/1 -> F(theta)/3(Theta)
  F(theta)/1(f_theta) -> Compare To Zero/1, Enabled Subsystem1/2(f_the)
  y/1 -> Divide2/2
  Divide2/1 -> Compare To Zero1/1
  Merge/1 -> "Proj(the, y)"/1
  "y "/1 -> Enabled Subsystem/1(In1)
  Enabled Subsystem/1(Out1) -> Merge/1
  Compare To Zero/1 -> Logical Operator2/2
  F(theta)/2(dif_f_theta) -> Divide2/1, Enabled Subsystem1/3(grad)
  Compare To Zero1/1 -> Logical Operator2/1
  Logical Operator2/1 -> Logical Operator/1, Enabled Subsystem1/Enable
  Logical Operator/1 -> Enabled Subsystem/Enable
  "y    "/1 -> Enabled Subsystem1/1(y)
  Enabled Subsystem1/1(Out1) -> Merge/2

== system controlMCUSlugsMKII/Inner Loop/ Navigation/L1 Output Feedback Controller With  Projection Operator/Protect NaNs ==
  In1 : Inport
  Integer Delay3 : simulink/Discrete/Integer Delay  Orientation=left  vinit=0.0  samptime=T  NumDelays=1
  Relational Operator2 : RelationalOperator  Operator===  LogicOutDataTypeMode=Specify via dialog
  Switch3 : Switch  Criteria=u2 > Threshold  Threshold=0.3  SampleTime=.01
  Out1 : Outport  Orientation=down
  wires:
  Relational Operator2/1 -> Switch3/2
  In1/1 -> Switch3/1, Relational Operator2/1, Relational Operator2/2
  Switch3/1 -> Integer Delay3/1, Out1/1
  Integer Delay3/1 -> Switch3/3

== system controlMCUSlugsMKII/Inner Loop/ Navigation/L1 Output Feedback Controller With  Projection Operator/Protect NaNs2 ==
  In1 : Inport
  Integer Delay3 : simulink/Discrete/Integer Delay  Orientation=left  vinit=0.0  samptime=T  NumDelays=1
  Relational Operator2 : RelationalOperator  Operator===  LogicOutDataTypeMode=Specify via dialog
  Switch3 : Switch  Criteria=u2 > Threshold  Threshold=0.3  SampleTime=.01
  Out1 : Outport  Orientation=down
  wires:
  Relational Operator2/1 -> Switch3/2
  In1/1 -> Switch3/1, Relational Operator2/1, Relational Operator2/2
  Switch3/1 -> Integer Delay3/1, Out1/1
  Integer Delay3/1 -> Switch3/3

== system controlMCUSlugsMKII/Inner Loop/ Navigation/L1 Output Feedback Controller With  Projection Operator/State Predictor ==
  a : Inport
  u : Inport  Port=2
  Compute Coef : Subsystem
  Detect Change : Subsystem
  Divide : Product  OutScaling=2^-10  SampleTime=apSampleTime
  Divide1 : Product  OutScaling=2^-10  SampleTime=apSampleTime
  IC : InitialCondition
  Integer Delay : simulink/Discrete/Integer Delay  vinit=0.0  samptime=apSampleTime  NumDelays=1
  Integer Delay1 : simulink/Discrete/Integer Delay  Orientation=left  vinit=0.0  samptime=apSampleTime  NumDelays=1
  Subtract : Sum  OutScaling=2^-10  SampleTime=apSampleTime
  y : Outport
  wires:
  Integer Delay1/1 -> Divide1/2
  u/1 -> Integer Delay/1
  IC/1 -> Compute Coef/Enable
  Subtract/1 -> Integer Delay1/1, y/1
  Divide1/1 -> Subtract/2
  Divide/1 -> Subtract/1
  Integer Delay/1 -> Divide/2
  Detect Change/1(change?) -> IC/1
  Compute Coef/2(c) -> Divide1/1
  Compute Coef/1(b) -> Divide/1
  a/1 -> Detect Change/1(Data), Compute Coef/1(a)

== system controlMCUSlugsMKII/Inner Loop/ Navigation/L1 Output Feedback Controller With  Projection Operator/Trapezoidal Integrator ==
  x : Inport
  Reset : Inport  Port=2
  Constant : Constant  Value=1/3  OutDataTypeMode=single
  Constant1 : Constant  Value=4/3  OutDataTypeMode=single
  Constant2 : Constant  Value=T/2  OutDataTypeMode=single
  Constant3 : Constant  Value=1/3  OutDataTypeMode=single
  Constant5 : Constant  Orientation=left  Value=0  OutDataTypeMode=single
  Integer Delay : simulink/Discrete/Integer Delay  vinit=0.0  samptime=T  NumDelays=1
  Integer Delay1 : simulink/Discrete/Integer Delay  vinit=0.0  samptime=T  NumDelays=2
  Integer Delay2 : simulink/Discrete/Integer Delay  Orientation=left  vinit=0.0  samptime=T  NumDelays=1
  Product{,1..3} (4 alike) : Product  OutDataTypeMode=single  RndMeth=Zero
  Protect NaNs : Subsystem
  Protect NaNs1 : Subsystem
  Subtract : Sum  Inputs=3  OutDataTypeMode=single  OutScaling=2^-10
  Subtract1 : Sum  Inputs=2  OutDataTypeMode=single  OutScaling=2^-10
  Switch1 : Switch  Criteria=u2 > Threshold  Threshold=0.3  SampleTime=.01
  "[min max]" : Saturate  UpperLimit=upperLimit  LowerLimit=lowerLimit  SampleTime=T
  Int(x) : Outport
  wires:
  Constant/1 -> Product/2
  Constant1/1 -> Product1/2
  Integer Delay/1 -> Product1/1
  Integer Delay1/1 -> Product2/1
  Constant3/1 -> Product2/2
  x/1 -> Protect NaNs/1(In1)
  Product/1 -> Subtract/1
  Product1/1 -> Subtract/2
  Product2/1 -> Subtract/3
  Constant2/1 -> Product3/1
  Subtract/1 -> Product3/2
  Integer Delay2/1 -> Subtract1/1
  Constant5/1 -> Switch1/1
  Reset/1 -> Switch1/2
  Switch1/1 -> Protect NaNs1/1(In1)
  "[min max]"/1 -> Switch1/3
  Product3/1 -> Subtract1/2
  Subtract1/1 -> "[min max]"/1
  Protect NaNs/1(Out1) -> Product/1, Integer Delay/1, Integer Delay1/1
  Protect NaNs1/1(Out1) -> Int(x)/1, Integer Delay2/1

== system controlMCUSlugsMKII/Inner Loop/ Navigation/Lateral Channel/0.5 sec  tau ==
  In1 : Inport
  Constant : Constant  Value=T
  Constant1 : Constant  Value=f
  Embedded MATLAB Function : Stateflow chart
  Out1 : Outport
  wires:
  Constant/1 -> Embedded MATLAB Function/2(T)
  Constant1/1 -> Embedded MATLAB Function/3(f)
  Embedded MATLAB Function/1(y) -> Out1/1
  In1/1 -> Embedded MATLAB Function/1(u)

== system controlMCUSlugsMKII/Inner Loop/ Navigation/Lateral Channel/Bank to Psi Dot ==
  phi_c : Inport
  U_m : Inport  Port=2
  Constant1 : Constant  Value=9.80665  OutDataTypeMode=single
  Divide : Product  Inputs=/*  OutDataTypeMode=single  OutScaling=2^-10
  Divide1 : Product  OutDataTypeMode=single  OutScaling=2^-10
  Protect NaNs : Subsystem
  Protect NaNs1 : Subsystem
  Subsystem8 : SLUGS_Library/Subsystem8  SystemSampleTime=-1
  "[0 40]" : Saturate  UpperLimit=40  LowerLimit=0  SampleTime=.01
  bank Limit : Saturate  UpperLimit=bankCommandLimit  LowerLimit=-bankCommandLimit  SampleTime=.01
  psi_dot_c : Outport
  wires:
  "[0 40]"/1 -> Divide/1
  Divide/1 -> Divide1/2
  phi_c/1 -> Protect NaNs/1(In1)
  Subsystem8/1 -> Divide1/1
  Divide1/1 -> psi_dot_c/1
  Constant1/1 -> Divide/2
  U_m/1 -> Protect NaNs1/1(In1)
  bank Limit/1 -> Subsystem8/1
  Protect NaNs/1(Out1) -> bank Limit/1
  Protect NaNs1/1(Out1) -> "[0 40]"/1

== system controlMCUSlugsMKII/Inner Loop/ Navigation/Lateral Channel/High Pass (Washout) Filter ==
  r : Inport
  Constant1 : Constant  Value=0.9992  OutDataTypeMode=single
  Constant2 : Constant  Orientation=left  Value=0.9983  OutDataTypeMode=single
  Constant3 : Constant  Value=0.9992  OutDataTypeMode=single
  Integer Delay : simulink/Discrete/Integer Delay  vinit=0.0  samptime=apSampleTime  NumDelays=1
  Integer Delay1 : simulink/Discrete/Integer Delay  Orientation=left  vinit=0.0  samptime=apSampleTime  NumDelays=1
  Product : Product  Orientation=left  RndMeth=Zero
  Product1 : Product  RndMeth=Zero
  Product2 : Product  RndMeth=Zero
  Subtract : Sum  Inputs=+-+  OutScaling=2^-10
  "[-2 2]" : Saturate  UpperLimit=2  LowerLimit=-2
  r_hp : Outport
  wires:
  r/1 -> Integer Delay/1, Product1/2
  Subtract/1 -> "[-2 2]"/1
  Integer Delay1/1 -> Product/1
  Constant2/1 -> Product/2
  Product/1 -> Subtract/3
  "[-2 2]"/1 -> r_hp/1, Integer Delay1/1
  Product1/1 -> Subtract/1
  Constant1/1 -> Product1/1
  Product2/1 -> Subtract/2
  Integer Delay/1 -> Product2/1
  Constant3/1 -> Product2/2

== system controlMCUSlugsMKII/Inner Loop/ Navigation/Lateral Channel/Protect NaNs ==
  In1 : Inport
  Integer Delay3 : simulink/Discrete/Integer Delay  Orientation=left  vinit=0.0  samptime=T  NumDelays=1
  Relational Operator2 : RelationalOperator  Operator===  LogicOutDataTypeMode=Specify via dialog
  Switch3 : Switch  Criteria=u2 > Threshold  Threshold=0.3  SampleTime=.01
  Out1 : Outport  Orientation=down
  wires:
  Relational Operator2/1 -> Switch3/2
  In1/1 -> Switch3/1, Relational Operator2/1, Relational Operator2/2
  Switch3/1 -> Integer Delay3/1, Out1/1
  Integer Delay3/1 -> Switch3/3

== system controlMCUSlugsMKII/Inner Loop/ Navigation/Lateral Channel/Protect NaNs1 ==
  In1 : Inport
  Integer Delay3 : simulink/Discrete/Integer Delay  Orientation=left  vinit=0.0  samptime=T  NumDelays=1
  Relational Operator2 : RelationalOperator  Operator===  LogicOutDataTypeMode=Specify via dialog
  Switch3 : Switch  Criteria=u2 > Threshold  Threshold=0.3  SampleTime=.01
  Out1 : Outport  Orientation=down
  wires:
  Integer Delay3/1 -> Switch3/3
  Switch3/1 -> Out1/1, Integer Delay3/1
  In1/1 -> Relational Operator2/2, Relational Operator2/1, Switch3/1
  Relational Operator2/1 -> Switch3/2

== system controlMCUSlugsMKII/Inner Loop/ Navigation/Lateral Channel/Protect NaNs2 ==
  In1 : Inport
  Integer Delay3 : simulink/Discrete/Integer Delay  Orientation=left  vinit=0.0  samptime=T  NumDelays=1
  Relational Operator2 : RelationalOperator  Operator===  LogicOutDataTypeMode=Specify via dialog
  Switch3 : Switch  Criteria=u2 > Threshold  Threshold=0.3  SampleTime=.01
  Out1 : Outport  Orientation=down
  wires:
  Relational Operator2/1 -> Switch3/2
  In1/1 -> Switch3/1, Relational Operator2/1, Relational Operator2/2
  Switch3/1 -> Integer Delay3/1, Out1/1
  Integer Delay3/1 -> Switch3/3

== system controlMCUSlugsMKII/Inner Loop/ Navigation/Lateral Channel/Protect NaNs3 ==
  In1 : Inport
  Integer Delay3 : simulink/Discrete/Integer Delay  Orientation=left  vinit=0.0  samptime=T  NumDelays=1
  Relational Operator2 : RelationalOperator  Operator===  LogicOutDataTypeMode=Specify via dialog
  Switch3 : Switch  Criteria=u2 > Threshold  Threshold=0.3  SampleTime=.01
  Out1 : Outport  Orientation=down
  wires:
  Integer Delay3/1 -> Switch3/3
  Switch3/1 -> Out1/1, Integer Delay3/1
  In1/1 -> Relational Operator2/2, Relational Operator2/1, Switch3/1
  Relational Operator2/1 -> Switch3/2

== system controlMCUSlugsMKII/Inner Loop/ Navigation/Lateral Channel/Sideslip Compensation ==
  phi_m : Inport
  r_m : Inport  Port=2
  U_m : Inport  Port=3
  Enable : EnablePort  StatesWhenEnabling=reset
  Bank to Psi Dot : Subsystem  AncestorBlock=SLUGS_Library/Navigation/Bank to Psi Dot
  Constant : Constant  Value=0.3  OutDataTypeMode=single
  Low Pass : Subsystem
      mask Display:
      | droots([],'-a','a')
      | port_label('input',1,'a')
      | port_label('input',2,'u')
      | port_label('output',1,'y')
  Protect NaNs2 : Subsystem
  Subtract : Sum  Inputs=+-  OutScaling=2^-10
  psi_dot to Bank : Subsystem  AncestorBlock=SLUGS_Library/Navigation/psi_dot to Bank
  bankComp : Outport  OutputWhenDisabled=reset  InitialOutput=0
  wires:
  Constant/1 -> Low Pass/1(a)
  Low Pass/1(y) -> bankComp/1
  psi_dot to Bank/1(phi_c) -> Protect NaNs2/1(In1)  "phi error"
  Subtract/1 -> psi_dot to Bank/1(psi_dot_c)  "turn rate error"
  Bank to Psi Dot/1(psi_dot_c) -> Subtract/1  "coord turn"
  U_m/1 -> psi_dot to Bank/2(U_m), Bank to Psi Dot/2(U_m)
  r_m/1 -> Subtract/2
  phi_m/1 -> Bank to Psi Dot/1(phi_c)
  Protect NaNs2/1(Out1) -> Low Pass/2(u)

== system controlMCUSlugsMKII/Inner Loop/ Navigation/Longitudinal Channel/0.3 sec  tau for low speeds ==
  In1 : Inport
  Constant : Constant  Value=T
  Constant1 : Constant  Value=f
  Embedded MATLAB Function : Stateflow chart
  Out1 : Outport
  wires:
  Constant/1 -> Embedded MATLAB Function/2(T)
  Constant1/1 -> Embedded MATLAB Function/3(f)
  Embedded MATLAB Function/1(y) -> Out1/1
  In1/1 -> Embedded MATLAB Function/1(u)

== system controlMCUSlugsMKII/Inner Loop/ Navigation/Longitudinal Channel/0.5 sec  tau for Turns ==
  In1 : Inport
  Constant : Constant  Value=T
  Constant1 : Constant  Value=f
  Embedded MATLAB Function : Stateflow chart
  Out1 : Outport
  wires:
  In1/1 -> Embedded MATLAB Function/1(u)
  Embedded MATLAB Function/1(y) -> Out1/1
  Constant1/1 -> Embedded MATLAB Function/3(f)
  Constant/1 -> Embedded MATLAB Function/2(T)

== system controlMCUSlugsMKII/Inner Loop/ Navigation/Longitudinal Channel/5 sec tau for high speeds ==
  In1 : Inport
  Constant : Constant  Value=T
  Constant1 : Constant  Value=f
  Embedded MATLAB Function : Stateflow chart
  Out1 : Outport
  wires:
  Constant/1 -> Embedded MATLAB Function/2(T)
  Constant1/1 -> Embedded MATLAB Function/3(f)
  Embedded MATLAB Function/1(y) -> Out1/1
  In1/1 -> Embedded MATLAB Function/1(u)

== system controlMCUSlugsMKII/Inner Loop/ Navigation/Longitudinal Channel/Air Density from Height ==
  h(m) : Inport
  Add : Sum  Inputs=+-  OutScaling=2^-10
  Constant : Constant  OutDataTypeMode=single
  Constant 2 from Model : Constant  Value=4.255876  OutDataTypeMode=single
  Constant from Model : Constant  Value=145442  OutDataTypeMode=single
  Divide : Product  Inputs=*/  OutScaling=2^-10
  Divide1 : Product  OutScaling=2^-10
  Length Conversion : aerolibconvert2/Length Conversion  SystemSampleTime=-1  IU=m  OU=ft
  Rho_0 (Kg/m^3) : Constant  Value=1.225  OutDataTypeMode=single
  Subsystem : Subsystem  AncestorBlock=SLUGS_Library/Subsystem
  "[0 1000]" : Saturate  UpperLimit=1000  LowerLimit=0
  rho (Kg/m^3) : Outport
  wires:
  Constant/1 -> Add/1
  Divide/1 -> Add/2
  h(m)/1 -> "[0 1000]"/1
  Constant from Model/1 -> Divide/2
  Rho_0 (Kg/m^3)/1 -> Divide1/2
  Divide1/1 -> rho (Kg/m^3)/1
  Length Conversion/1 -> Divide/1
  Add/1 -> Subsystem/1(u)
  Constant 2 from Model/1 -> Subsystem/2(v)
  Subsystem/1(u^v) -> Divide1/1
  "[0 1000]"/1 -> Length Conversion/1

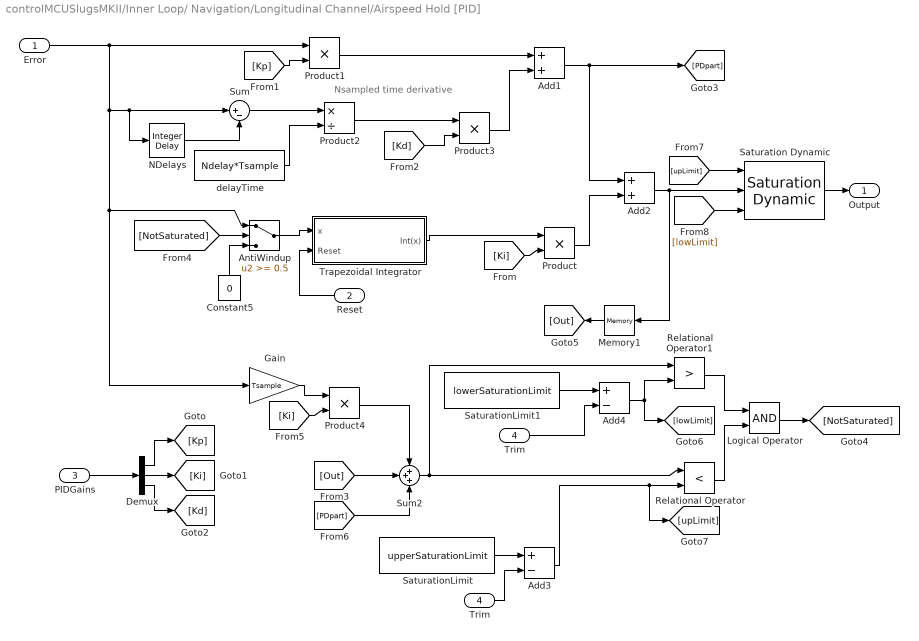
== system controlMCUSlugsMKII/Inner Loop/ Navigation/Longitudinal Channel/Airspeed Hold [PID] ==
  note: Nsampled time derivative
  Error : Inport
  Reset : Inport  Orientation=left  Port=2
  PIDGains : Inport  Port=3
  Trim : Inport  Port=4
  Add1 : Sum  OutScaling=2^-10
  Add2 : Sum  OutDataTypeMode=single  OutScaling=2^-10
  Add3 : Sum  Inputs=+-  OutDataTypeMode=single  OutScaling=2^-10
  Add4 : Sum  Inputs=+-  OutDataTypeMode=single  OutScaling=2^-10
  AntiWindup : Switch  Threshold=0.5
  Constant5 : Constant  Orientation=up  Value=0  OutDataTypeMode=double
  Demux : Demux  Outputs=3
  Gain : Gain  Gain=Tsample
  Logical Operator : Logic  AllPortsSameDT=off  OutDataTypeMode=Boolean
  Memory1 : Memory  Orientation=left  InheritSampleTime=on
  NDelays : simulink/Discrete/Integer Delay  vinit=0.0  samptime=Tsample  NumDelays=Ndelay
  Product{,1,3..4} (4 alike) : Product  RndMeth=Zero
  Product2 : Product  Inputs=*/  RndMeth=Zero
  Relational Operator : RelationalOperator  Operator=<  LogicOutDataTypeMode=Boolean
  Relational Operator1 : RelationalOperator  Operator=>  LogicOutDataTypeMode=Boolean
  Saturation Dynamic : simulink/Discontinuities/Saturation Dynamic  SystemSampleTime=-1
  SaturationLimit : Constant  Value=upperSaturationLimit  OutDataTypeMode=single
  SaturationLimit1 : Constant  Value=lowerSaturationLimit  OutDataTypeMode=single
  Sum : Sum  Inputs=|+-
  Sum2 : Sum  Inputs=+++
  Trapezoidal Integrator : Subsystem  mask{T=Tsample}
      mask prompts: T "Sample Time"
  "Trim " : InportShadow  Port=4  LatchByCopyingInsideSignal=off
  delayTime : Constant  Value=Ndelay*Tsample  OutDataTypeMode=single
  Output : Outport
  wires:
  [lowLimit] -> Saturation Dynamic/3
  [upLimit] -> Saturation Dynamic/1
  "Trim "/1 -> Add4/2
  SaturationLimit1/1 -> Add4/1
  Add4/1 -> [lowLimit], Relational Operator1/2
  SaturationLimit/1 -> Add3/1
  Trim/1 -> Add3/2
  Logical Operator/1 -> [NotSaturated]
  Relational Operator1/1 -> Logical Operator/1
  Relational Operator/1 -> Logical Operator/2
  Add3/1 -> [upLimit], Relational Operator/2
  [Out] -> Sum2/2
  Sum2/1 -> Relational Operator1/1, Relational Operator/1
  [Ki] -> Product4/2
  Gain/1 -> Product4/1
  Product4/1 -> Sum2/1
  [PDpart] -> Sum2/3
  Product/1 -> Add2/2
  Add1/1 -> Add2/1, [PDpart]
  Product3/1 -> Add1/2
  Product1/1 -> Add1/1
  Reset/1 -> Trapezoidal Integrator/2(Reset)
  Memory1/1 -> [Out]
  PIDGains/1 -> Demux/1
  Demux/1 -> [Kp]
  Demux/2 -> [Ki]
  Demux/3 -> [Kd]
  Constant5/1 -> AntiWindup/3
  AntiWindup/1 -> Trapezoidal Integrator/1(x)
  Error/1 -> Gain/1, AntiWindup/1, NDelays/1, Sum/1, Product1/1
  [Ki] -> Product/2
  Trapezoidal Integrator/1(Int(x)) -> Product/1
  [Kp] -> Product1/2
  Add2/1 -> Saturation Dynamic/2, Memory1/1
  NDelays/1 -> Sum/2
  Sum/1 -> Product2/1
  delayTime/1 -> Product2/2
  [Kd] -> Product3/2
  Product2/1 -> Product3/1
  Saturation Dynamic/1 -> Output/1
  [NotSaturated] -> AntiWindup/2

== system controlMCUSlugsMKII/Inner Loop/ Navigation/Longitudinal Channel/Compute Airspeed ==
  Dyn P : Inport
  rho : Inport  Port=2
  Divide2 : Product  Inputs=**/  OutScaling=2^-10
  Subsystem1 : Subsystem  AncestorBlock=SLUGS_Library/Subsystem1
  "[ 0.01 50000]" : Saturate  UpperLimit=50000  LowerLimit=0.01
  a : Constant  Value=2  OutDataTypeMode=single
  Airspeed m(s) : Outport
  wires:
  "[ 0.01 50000]"/1 -> Divide2/3
  rho/1 -> "[ 0.01 50000]"/1
  Dyn P/1 -> Divide2/2
  a/1 -> Divide2/1
  Subsystem1/1(sqrt(x)) -> Airspeed m(s)/1
  Divide2/1 -> Subsystem1/1(x)
